simulink model "RC_BOT"  (Simulink 9.2)
settings: Solver=ode1  StartTime=0.0  StopTime=50000  FixedStep=0.1  RelTol=1e-3  EnableMultiTasking=on
settings Model: Creator=user  LastModifiedBy=user
settings DataIOCC: SignalLoggingSaveFormat=Dataset
settings DebuggingCC: UnderspecifiedInitializationDetection=Simplified  MergeDetectMultiDrivingBlocksExec=error  SolverPrmCheckMsg=warning  FcnCallInpInsideContextMsg=error  StateNameClashWarn=none
settings GRTTargetCC: CombineOutputUpdateFcns=on  GRTInterface=off
settings ConfigComp: CovSFcnEnable=off

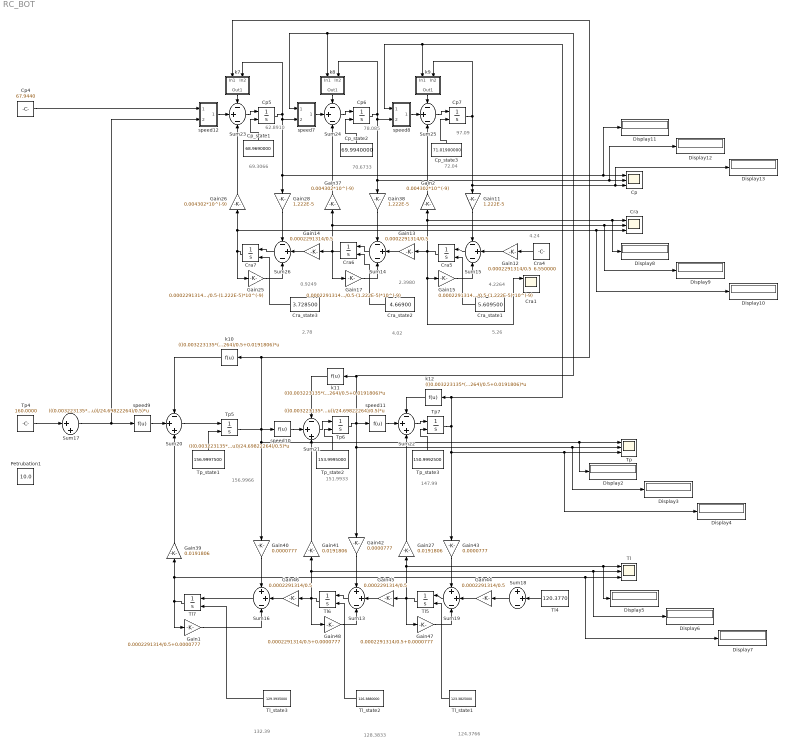
== system RC_BOT ==
  note: 0.9249
  note: 2.3980
  note: 4.2264
  note: 62.8910
  note: 78.085
  note: 97.09
  note: 2.78
  note: 4.02
  note: 5.26
  note: 72.04
  note: 70.6733
  note: 69.3066
  note: 132.39
  note: 128.3833
  note: 124.3766
  note: 147.99
  note: 151.9933
  note: 156.9966
  note: 4.24
  Cp : Scope  NumInputPorts=3
  Cp4 : Constant  Value=67.9440
  Cp5 : Integrator  InitialConditionSource=external  InitialCondition=69.3066
  Cp6 : Integrator  InitialConditionSource=external  InitialCondition=70.6733
  Cp7 : Integrator  InitialConditionSource=external  InitialCondition=72.04
  Cp_state1 : Constant  Value=68.9690000
  Cp_state2 : Constant  Value=69.9940000
  Cp_state3 : Constant  Value=71.01900000
  Cra : Scope  NumInputPorts=3
  Cra1 : Scope  NumInputPorts=3
  Cra4 : Constant  Value=6.550000
  Cra5 : Integrator  InitialConditionSource=external  InitialCondition=5.26
  Cra6 : Integrator  InitialConditionSource=external  InitialCondition=4.02
  Cra7 : Integrator  InitialConditionSource=external  InitialCondition=2.78
  Cra_state1 : Constant  Value=5.609500
  Cra_state2 : Constant  Value=4.66900
  Cra_state3 : Constant  Value=3.728500
  Display{2..13} (12 alike) : Display
  Gain1 : Gain  Gain=0.0002291314/0.5+0.0000777
  Gain11 : Gain  Gain=1.222E-5
  Gain{12..14,44..46} (6 alike) : Gain  Gain=0.0002291314/0.5
  Gain15 : Gain  Gain=0.0002291314/0.5-(1.222E-5)*10^(-9)
  Gain17 : Gain  Gain=0.0002291314/0.5-(1.222E-5)*10^(-9)
  Gain2 : Gain  Gain=0.004302*10^(-9)
  Gain25 : Gain  Gain=0.0002291314/0.5-(1.222E-5)*10^(-9)
  Gain26 : Gain  Gain=0.004302*10^(-9)
  Gain27 : Gain  Gain=0.0191806
  Gain28 : Gain  Gain=1.222E-5
  Gain37 : Gain  Gain=0.004302*10^(-9)
  Gain38 : Gain  Gain=1.222E-5
  Gain39 : Gain  Gain=0.0191806
  Gain40 : Gain  Gain=0.0000777
  Gain41 : Gain  Gain=0.0191806
  Gain42 : Gain  Gain=0.0000777
  Gain43 : Gain  Gain=0.0000777
  Gain47 : Gain  Gain=0.0002291314/0.5+0.0000777
  Gain48 : Gain  Gain=0.0002291314/0.5+0.0000777
  Petrubation1 : Constant  Value=10.0
  Sum{13,16,18..19} (4 alike) : Sum  Inputs=++-
  Sum{14..15,23..26} (6 alike) : Sum  Inputs=-+-
  Sum17 : Sum  Inputs=|++
  Sum20 : Sum  Inputs=-++
  Sum21 : Sum  Inputs=-++
  Sum22 : Sum  Inputs=-++
  Tl : Scope  NumInputPorts=3
  Tl4 : Constant  Value=120.3770
  Tl5 : Integrator  InitialConditionSource=external  InitialCondition=124.3766
  Tl6 : Integrator  InitialConditionSource=external  InitialCondition=128.3833
  Tl7 : Integrator  InitialConditionSource=external  InitialCondition=132.39
  "Tl_state1 " : Constant  Value=123.3825000
  Tl_state2 : Constant  Value=126.3880000
  Tl_state3 : Constant  Value=129.3935000
  Tp : Scope  NumInputPorts=3
  Tp4 : Constant  Value=160.0000
  Tp5 : Integrator  InitialConditionSource=external  InitialCondition=156.9966
  Tp6 : Integrator  InitialConditionSource=external  InitialCondition=151.9933
  Tp7 : Integrator  InitialConditionSource=external  InitialCondition=147.99  IgnoreLimit=on
  Tp_state1 : Constant  Value=156.9997500
  Tp_state2 : Constant  Value=153.9995000
  Tp_state3 : Constant  Value=150.9992500
  k10 : Fcn  Expr=(((0.003223135*(273+u))/24.69822264)/0.5+0.0191806)*u
  k11 : Fcn  Expr=(((0.003223135*(273+u))/24.69822264)/0.5+0.0191806)*u
  k12 : Fcn  Expr=(((0.003223135*(273+u))/24.69822264)/0.5+0.0191806)*u
  k7 : Subsystem
  k8 : Subsystem
  k9 : Subsystem
  speed10 : Fcn  Expr=(((0.003223135*(273+u))/24.69822264)/0.5)*u
  speed11 : Fcn  Expr=(((0.003223135*(273+u))/24.69822264)/0.5)*u
  speed12 : Subsystem
  speed7 : Subsystem
  speed8 : Subsystem
  speed9 : Fcn  Expr=(((0.003223135*(273+u))/24.69822264)/0.5)*u
  wires:
  Sum23/1 -> Cp5/1
  speed7/1(Out1) -> Sum24/2
  Sum24/1 -> Cp6/1
  speed8/1(Out1) -> Sum25/2
  Sum25/1 -> Cp7/1
  Cp5/1 -> speed7/2(In2), Gain28/1, Cp/1, Display11/1, k7/2(In2)
  Gain26/1 -> Sum23/3
  Cp7/1 -> k9/2(In2), Gain11/1, Display13/1, Cp/3
  Gain37/1 -> Sum24/3
  Gain2/1 -> Sum25/3
  Gain28/1 -> Sum26/1
  Gain38/1 -> Sum14/1
  Gain11/1 -> Sum15/1
  Gain12/1 -> Sum15/2
  Sum15/1 -> Cra5/1
  Cra5/1 -> Cra1/1, Gain15/1, Gain13/1, Gain2/1, Display8/1, Cra/1
  Gain13/1 -> Sum14/2
  Sum14/1 -> Cra6/1
  Gain14/1 -> Sum26/2
  Sum26/1 -> Cra7/1
  Gain15/1 -> Sum15/3
  Gain17/1 -> Sum14/3
  Gain25/1 -> Sum26/3
  speed9/1 -> Sum20/2
  k10/1 -> Sum20/1
  Sum20/1 -> Tp5/1
  speed10/1 -> Sum21/2
  k11/1 -> Sum21/1
  Sum21/1 -> Tp6/1
  speed11/1 -> Sum22/2
  k12/1 -> Sum22/1
  Sum22/1 -> Tp7/1
  Gain39/1 -> Sum20/3
  Gain41/1 -> Sum21/3
  Gain27/1 -> Sum22/3
  Gain40/1 -> Sum16/1
  Gain42/1 -> Sum13/1
  Gain43/1 -> Sum19/1
  Gain44/1 -> Sum19/2
  Sum19/1 -> Tl5/1
  Tl5/1 -> Gain47/1, Gain45/1, Gain27/1, Display5/1, Tl/1
  Gain45/1 -> Sum13/2
  Sum13/1 -> Tl6/1
  Gain46/1 -> Sum16/2
  Sum16/1 -> Tl7/1
  Gain47/1 -> Sum19/3
  Gain48/1 -> Sum13/3
  Gain1/1 -> Sum16/3
  speed12/1(Out1) -> Sum23/2
  Cp4/1 -> speed12/1(In1)
  k7/1(Out1) -> Sum23/1
  k8/1(Out1) -> Sum24/1
  k9/1(Out1) -> Sum25/1
  Cra4/1 -> Gain12/1
  Sum17/1 -> speed9/1, speed12/2(In2)
  Sum18/1 -> Gain44/1
  Tp4/1 -> Sum17/1
  Tl4/1 -> Sum18/2
  Tp6/1 -> Gain42/1, Display3/1, Tp/2, k11/1, speed7/1(In1), k8/1(In1), speed11/1
  Tp5/1 -> Gain40/1, Display2/1, Tp/1, k10/1, k7/1(In1), speed10/1
  Tp_state1/1 -> Tp5/2
  Tp_state3/1 -> Tp7/2
  "Tl_state1 "/1 -> Tl5/2
  Tl_state2/1 -> Tl6/2
  Tl_state3/1 -> Tl7/2
  Cp_state1/1 -> Cp5/2
  Cp_state2/1 -> Cp6/2
  Cp_state3/1 -> Cp7/2
  Cra_state1/1 -> Cra5/2
  Cra_state2/1 -> Cra6/2
  Cra_state3/1 -> Cra7/2
  Tp_state2/1 -> Tp6/2
  Tl6/1 -> Gain48/1, Gain46/1, Gain41/1, Display6/1, Tl/2
  Tl7/1 -> Gain1/1, Gain39/1, Display7/1, Tl/3
  Cra6/1 -> Gain17/1, Gain14/1, Gain37/1, Display9/1, Cra/2
  Cra7/1 -> Gain25/1, Gain26/1, Display10/1, Cra/3
  Cp6/1 -> speed8/2(In2), Gain38/1, Display12/1, Cp/2, k8/2(In2)
  Tp7/1 -> Gain43/1, Display4/1, Tp/3, k9/1(In1), speed8/1(In1), k12/1

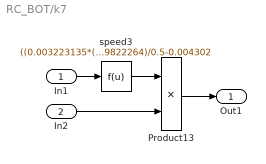
== system RC_BOT/k7 ==
  In1 : Inport
  In2 : Inport  Port=2
  Product13 : Product  SaturateOnIntegerOverflow=on  InputSameDT=on  OutDataTypeStr=Inherit: Same as first input
  speed3 : Fcn  Expr=((0.003223135*(273+u))/24.69822264)/0.5-0.004302
  Out1 : Outport
  wires:
  Product13/1 -> Out1/1
  speed3/1 -> Product13/1
  In1/1 -> speed3/1
  In2/1 -> Product13/2

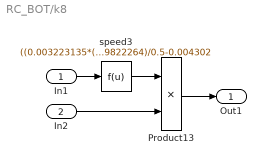
== system RC_BOT/k8 ==
  In1 : Inport
  In2 : Inport  Port=2
  Product13 : Product  SaturateOnIntegerOverflow=on  InputSameDT=on  OutDataTypeStr=Inherit: Same as first input
  speed3 : Fcn  Expr=((0.003223135*(273+u))/24.69822264)/0.5-0.004302
  Out1 : Outport
  wires:
  Product13/1 -> Out1/1
  speed3/1 -> Product13/1
  In1/1 -> speed3/1
  In2/1 -> Product13/2

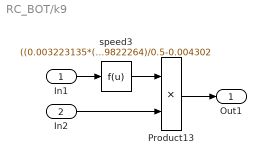
== system RC_BOT/k9 ==
  In1 : Inport
  In2 : Inport  Port=2
  Product13 : Product  SaturateOnIntegerOverflow=on  InputSameDT=on  OutDataTypeStr=Inherit: Same as first input
  speed3 : Fcn  Expr=((0.003223135*(273+u))/24.69822264)/0.5-0.004302
  Out1 : Outport
  wires:
  Product13/1 -> Out1/1
  speed3/1 -> Product13/1
  In1/1 -> speed3/1
  In2/1 -> Product13/2

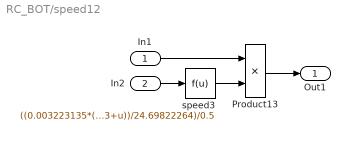
== system RC_BOT/speed12 ==
  In1 : Inport
  In2 : Inport  Port=2
  Product13 : Product  SaturateOnIntegerOverflow=on  InputSameDT=on  OutDataTypeStr=Inherit: Same as first input
  speed3 : Fcn  Expr=((0.003223135*(273+u))/24.69822264)/0.5
  Out1 : Outport
  wires:
  In1/1 -> Product13/1
  In2/1 -> speed3/1
  speed3/1 -> Product13/2
  Product13/1 -> Out1/1

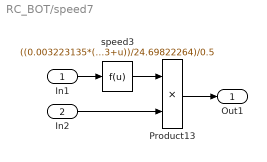
== system RC_BOT/speed7 ==
  In1 : Inport
  In2 : Inport  Port=2
  Product13 : Product  SaturateOnIntegerOverflow=on  InputSameDT=on  OutDataTypeStr=Inherit: Same as first input
  speed3 : Fcn  Expr=((0.003223135*(273+u))/24.69822264)/0.5
  Out1 : Outport
  wires:
  Product13/1 -> Out1/1
  In2/1 -> Product13/2
  speed3/1 -> Product13/1
  In1/1 -> speed3/1

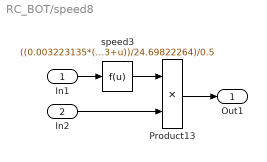
== system RC_BOT/speed8 ==
  In1 : Inport
  In2 : Inport  Port=2
  Product13 : Product  SaturateOnIntegerOverflow=on  InputSameDT=on  OutDataTypeStr=Inherit: Same as first input
  speed3 : Fcn  Expr=((0.003223135*(273+u))/24.69822264)/0.5
  Out1 : Outport
  wires:
  Product13/1 -> Out1/1
  In2/1 -> Product13/2
  speed3/1 -> Product13/1
  In1/1 -> speed3/1
